simulink model "si3b_coilDC"  (R2024a)
settings: Solver=VariableStepAuto  StartTime=0.0  StopTime=te(2)  RelTol=1e-3
values from neighbouring files (symbols this model uses):
  L = 44.15e-3    (= 0.04415)    [Electromagnet_par.m]    (also in coil_ironcore.m = 1; sim21_ODE.m = 1)
  R = 6.5    [Electromagnet_par.m]    (also in coil_ironcore.m = 10; sim21_ODE.m = 10)
  U = 10    [Electromagnet_par.m]    (also in coil_ironcore.m = 163; sim21_ODE.m = 230*sqrt(2))
settings Model: Creator=ocean  LastModifiedBy=ocean

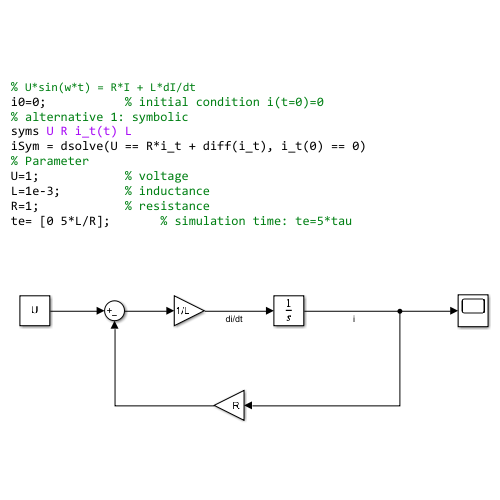
[thumbnail: Simulink's stored preview of the top-level diagram]
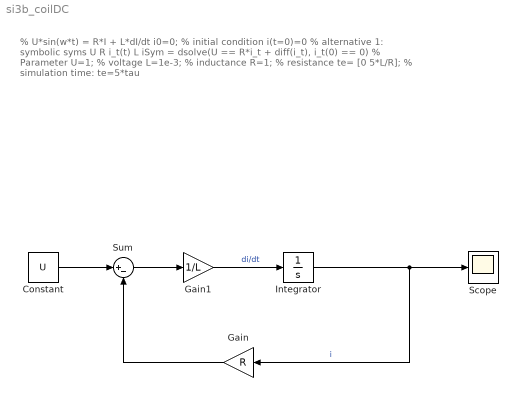
== system si3b_coilDC ==
  note: % U*sin(w*t) = R*I + L*dI/dt
      | i0=0; % initial condition i(t=0)=0
      | % alternative 1: symbolic
      | syms U R i_t(t) L
      | iSym = dsolve(U == R*i_t + diff(i_t), i_t(0) == 0)
      | % Parameter
      | U=1; % voltage
      | L=1e-3; % inductance
      | R=1; % resistance
      | te= [0 5*L/R]; % simulation time: te=5*tau
  Constant : Constant  Value=U
  Gain : Gain  Gain=R
  Gain1 : Gain  Gain=1/L
  Integrator : Integrator
  Scope : Scope
  Sum : Sum  Inputs=|+-
  wires:
  Integrator/1 -> Gain/1, Scope/1  "i"
  Constant/1 -> Sum/1
  Sum/1 -> Gain1/1
  Gain1/1 -> Integrator/1  "di/dt"
  Gain/1 -> Sum/2
